simulink model "robot_sim_TamePID_separated_FeedForward"  (R2025b)
settings: Solver=VariableStepAuto  StartTime=0.0  StopTime=80  RelTol=1e-3
settings Model: Creator=sjoer  LastModifiedBy=Ricardo Díaz

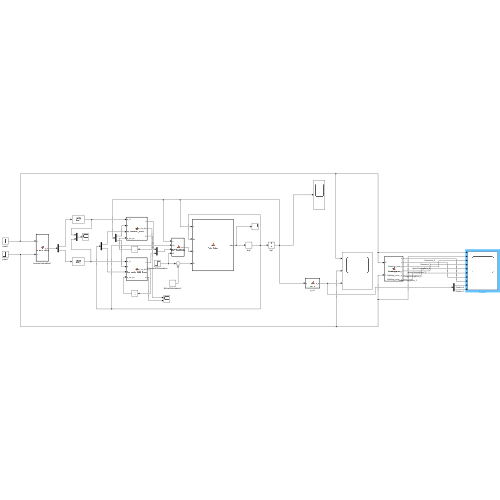
[thumbnail: Simulink's stored preview of the top-level diagram]
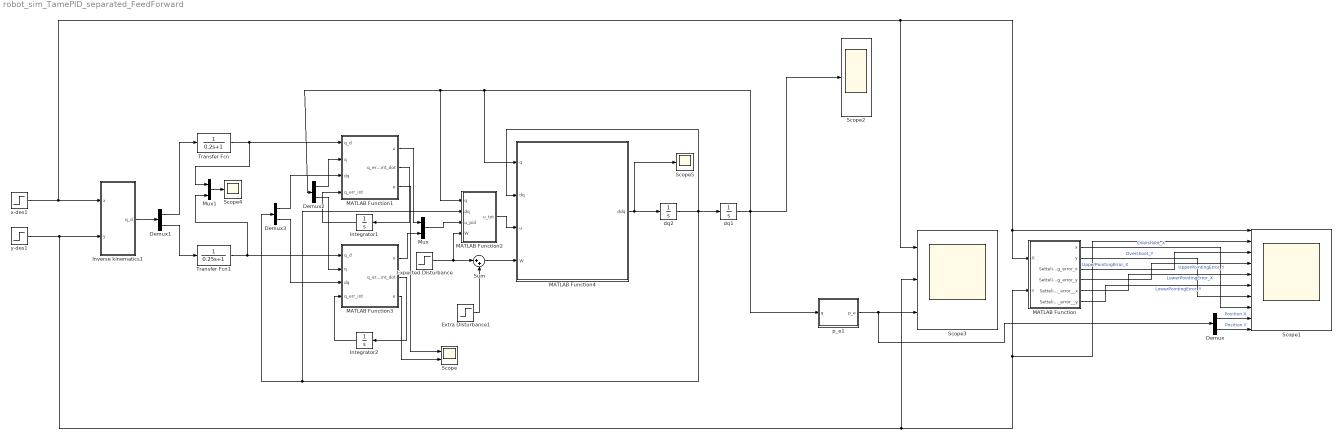
== system robot_sim_TamePID_separated_FeedForward ==
  Demux{,1..3} (4 alike) : Demux  Outputs=2
  Expected Disturbance : Step  Time=20  After=[60;0]  SampleTime=0
  Extra Disturbance1 : Step  Time=40  After=[1;0]  SampleTime=0
  Integrator1 : Integrator
  Integrator2 : Integrator
  Inverse kinematics1 : MATLAB Function  TreatAsAtomicUnit=on
  MATLAB Function : MATLAB Function  TreatAsAtomicUnit=on
  MATLAB Function1 : MATLAB Function  TreatAsAtomicUnit=on
  MATLAB Function2 : MATLAB Function  TreatAsAtomicUnit=on
  MATLAB Function3 : MATLAB Function  TreatAsAtomicUnit=on
  MATLAB Function4 : MATLAB Function  TreatAsAtomicUnit=on
  Mux : Mux  Inputs=2
  Mux1 : Mux  Inputs=2
  Scope : Scope  NumInputPorts=2
      settings: ActiveDisplayYMinimum=-0.18091547837897987  ActiveDisplayYMaximum=0.77180614923452828
  Scope1 : Scope  NumInputPorts=10
      settings: ActiveDisplayYMinimum=-0.015396490641404637  ActiveDisplayYMaximum=0.38455420077675151
  Scope2 : Scope
      settings: ActiveDisplayYMinimum=-1.4051776468584192  ActiveDisplayYMaximum=7.2505527137627759  DataLoggingVariableName=ScopeData2
  Scope3 : Scope  NumInputPorts=3
      settings: ActiveDisplayYMinimum=-0.23475497990891953  ActiveDisplayYMaximum=1.1640283494575223  DataLoggingVariableName=ScopeData3
  Scope4 : Scope
      settings: ActiveDisplayYMinimum=0.84247118511074626  ActiveDisplayYMaximum=1.1179895201691603  DataLoggingVariableName=ScopeData4
  Scope5 : Scope
      settings: ActiveDisplayYMinimum=-1  ActiveDisplayYMaximum=1  DataLoggingVariableName=ScopeData5
  Sum : Sum  Inputs=|++
  Transfer Fcn : TransferFcn  Denominator=[0.2 1]
  Transfer Fcn1 : TransferFcn  Denominator=[0.25 1]
  dq1 : Integrator
  dq2 : Integrator
  p_e1 : MATLAB Function  TreatAsAtomicUnit=on
  x-des1 : Step  Time=2  After=0.985  SampleTime=0
  y-des1 : Step  Time=2  After=0.174  SampleTime=0
  wires:
  Inverse kinematics1/1(q_d) -> Demux1/1
  Demux1/1 -> Transfer Fcn/1
  Demux1/2 -> Transfer Fcn1/1
  MATLAB Function4/1(ddq) -> Scope5/1, dq2/1
  dq2/1 -> MATLAB Function4/2(dq), MATLAB Function2/2(dq), Demux3/1, dq1/1
  x-des1/1 -> Scope3/1, MATLAB Function/1(X), Scope1/1, Inverse kinematics1/1(x)
  y-des1/1 -> Scope3/2, MATLAB Function/2(Y), Scope1/2, Inverse kinematics1/2(y)
  Demux2/1 -> MATLAB Function1/2(q)
  Demux2/2 -> MATLAB Function3/2(q)
  MATLAB Function1/1(u) -> Mux/1
  MATLAB Function3/1(u) -> Mux/2
  Integrator1/1 -> MATLAB Function1/4(q_err_int)
  MATLAB Function3/2(q_err_int_dot) -> Integrator2/1
  Integrator2/1 -> MATLAB Function3/4(q_err_int)
  Demux3/1 -> MATLAB Function1/3(dq)
  Demux3/2 -> MATLAB Function3/3(dq)
  Expected Disturbance/1 -> Sum/1, MATLAB Function2/4(W)
  dq1/1 -> MATLAB Function4/1(q), MATLAB Function2/1(q), Demux2/1, Scope2/1, p_e1/1(q)
  MATLAB Function1/2(q_err_int_dot) -> Integrator1/1
  Mux/1 -> MATLAB Function2/3(u_pid)
  MATLAB Function2/1(u_tot) -> MATLAB Function4/3(u)
  Transfer Fcn1/1 -> Mux1/2, MATLAB Function3/1(q_d)
  Transfer Fcn/1 -> Mux1/1, MATLAB Function1/1(q_d)
  MATLAB Function/3(Setteling_error_x) -> Scope1/3  "UpperPointingError_X"
  MATLAB Function/4(Setteling_error_y) -> Scope1/4  "UpperPointingError_Y"
  MATLAB Function/5(Setteling_error__x) -> Scope1/5  "LowerPointingError_X"
  MATLAB Function/6(Setteling_error__y) -> Scope1/6  "LowerPointingError_Y"
  MATLAB Function/2(y) -> Scope1/7  "Overshoot_Y"
  MATLAB Function/1(x) -> Scope1/8  "Overshoot_X"
  p_e1/1(p_e) -> Demux/1, Scope3/3
  Sum/1 -> MATLAB Function4/4(W)
  Extra Disturbance1/1 -> Sum/2
  Demux/1 -> Scope1/9  "Position X"
  Demux/2 -> Scope1/10  "Position Y"
  MATLAB Function3/3(e) -> Scope/2
  MATLAB Function1/3(e) -> Scope/1
  Mux1/1 -> Scope4/1

== matlab function robot_sim_TamePID_separated_FeedForward/MATLAB Function2 ==
  data: q input; dq input; u_pid input; W input; u_tot output
function u_tot = PolarFeedforward(q, dq, u_pid, W)
% --- Robot Parameters ---
I1 = 1.5; 
I2 = 0.5; 
l_c1 = 0.5;
m1 = 15;
m2 = 8;
g = 9.81;
alpha = -pi/2;

q1 = q(1);
q2 = q(2);
dq1 = dq(1);
dq2 = dq(2);

% Coriolis
c = [2*dq1*dq2*m2*q2;
    -(dq1^2)*m2*q2];

% Gravity
G = [g*cos(alpha - q1)*(l_c1*m1 + m2*q2);
    -g*m2*sin(alpha - q1)];

% J(q) - Jacobian
J = [-q2*sin(q1), cos(q1);
      q2*cos(q1), sin(q1)];

% Feedforward term
u_ff = c + G - J'*W;

u_tot = u_pid + u_ff;

end

== matlab function robot_sim_TamePID_separated_FeedForward/MATLAB Function ==
  data: x output; X input; y output; Y input; Setteling_error_x output; Setteling_error_y output; Setteling_error__x output; Setteling_error__y output
function [x,y,Setteling_error_x,Setteling_error_y,Setteling_error__x,Setteling_error__y] = OvershootLine(X,Y)

y = Y + Y*0.1;
x = X+X*0.1;
Setteling_error_x = X+X*0.02;
Setteling_error_y = Y + Y*0.02;

Setteling_error__x = X-X*0.02;
Setteling_error__y = Y -Y*0.02;

== matlab function robot_sim_TamePID_separated_FeedForward/MATLAB Function1 ==
  data: q_d input size=1 1; u output size=1 1; q input size=1 1; dq input size=1 1; q_err_int input size=1 1; q_err_int_dot output; e output
function [u, q_err_int_dot,e] = JointPID_Tame(q_d, q, dq, q_err_int)

%Initial values:

u_min=-6;
u_max= 6;
Ti=6;

% Rotation Joint (q1)
Kp1 = 120;
Kd1 = 100;
Ki1 = 1.5;

e = q_d - q;                                %Error

q_err_int_dot = e - (1/Ti)*q_err_int;       %Tamed integral

u_unsat = Kp1*e + Ki1*q_err_int - Kd1*dq;   %Unsaturated control

u = min(max(u_unsat, u_min), u_max);        %Saturation

if u ~= u_unsat
    q_err_int_dot = 0;                      %Anti Windup
end

end


%{
function [u,e] = JointPID(q_d, q, dq, q_err_int, Kp1, Ki1, Kd1) 
% Scalar joint PID controller 
% Error 
e = q_d - q; 
% Joint 1 (Rotation) 
u = (Kp1 * e) + (Ki1 * q_err_int) - (Kd1 * dq); %tau 
end
%}

== matlab function robot_sim_TamePID_separated_FeedForward/MATLAB Function3 ==
  data: q_d input size=1 1; u output size=1 1; q input size=1 1; dq input size=1 1; q_err_int input size=1 1; q_err_int_dot output size=1 1; e output
function [u, q_err_int_dot,e] = TranslationPID_Tame(q_d, q, dq, q_err_int)

%Initial values:

u_min=-75;
u_max= 75;
Ti=4;

% Prismatic Joint (q2)
Kp2 = 100;
Kd2 = 105;
Ki2 = 1.5;

e = q_d - q;                                %Error

q_err_int_dot = e - (1/Ti)*q_err_int;       %Tamed integral

u_unsat = Kp2*e + Ki2*q_err_int - Kd2*dq;   %Unsaturated control

u = min(max(u_unsat, u_min), u_max);        %Saturation

if u ~= u_unsat
    q_err_int_dot = 0;                      %Anti Windup
end

end
%{
function [u,e] = TranslationPID(q_d, q, dq, q_err_int, Kp2, Ki2, Kd2)
% Scalar joint PID controller

% Error
e = q_d - q;

% Joint 2 (Prismatic)
u = (Kp2 * e) + (Ki2 * q_err_int) - (Kd2 * dq); %F
end
%}

== matlab function robot_sim_TamePID_separated_FeedForward/Inverse kinematics1 ==
  data: x input; q_d output size=2 1; y input
function q_d  = InverseKinematics(x, y)
    % This block runs every time step
    
    % Extension (Prismatic Joint)
    q2_d = sqrt(x^2 + y^2);
    
    % Rotation (Revolute Joint)
    % We use atan2 to handle all quadrants automatically
    q1_d = atan2(y, x);

    q_d = [q1_d; q2_d];
end

== matlab function robot_sim_TamePID_separated_FeedForward/MATLAB Function4 ==
  data: q input; ddq output; dq input; u input; W input
function ddq  = PolarRobot(q, dq, u, W)
% Only the dynamic equations remain here

% --- Robot Parameters ---
I1 = 1.5; 
I2 = 0.5; 
l_c1 = 0.5;
m1 = 15;
m2 = 8;
g = 9.81;
alpha = -pi/2;

% --- Damping ---
d1 = 2.0; 
d2 = 5.0; 
D = [d1 0; 0 d2];

% --- Control / Simulation Setup ---
S = eye(2);

% Vectors
q1 = q(1);
q2 = q(2);
dq_1 = dq(1);
dq_2 = dq(2);

% M(q) - Mass matrix (Changes with q2)
M = [I1 + I2 + (l_c1^2)*m1 + m2*(q2^2), 0;
     0, m2];

% c(q,dq) - Coriolis (Changes with q2, dq1, dq2)
c = [2*dq_1*dq_2*m2*q2;
    -(dq_1^2)*m2*q2];

% G(q) - Gravity (Changes with q1, q2)
G = [g*cos(alpha - q1)*(l_c1*m1 + m2*q2);
    -g*m2*sin(alpha - q1)];

% J(q) - Jacobian
J = [-q2*sin(q1), cos(q1);
      q2*cos(q1), sin(q1)];

% Solving for ddq
ddq = M \ (S*u + J'* W - c - D*dq - G);

== matlab function robot_sim_TamePID_separated_FeedForward/p_e1 ==
  data: q input; p_e output
function p_e = ee_p(q)

p_e = [q(2)*cos(q(1)); q(2)*sin(q(1))];
